simulink model "practica15sim"  (R2015a)
settings: Solver=ode45  StartTime=0.0  StopTime=30  RelTol=1e-3
settings Model: Creator=Sala8  LastModifiedBy=Sala7

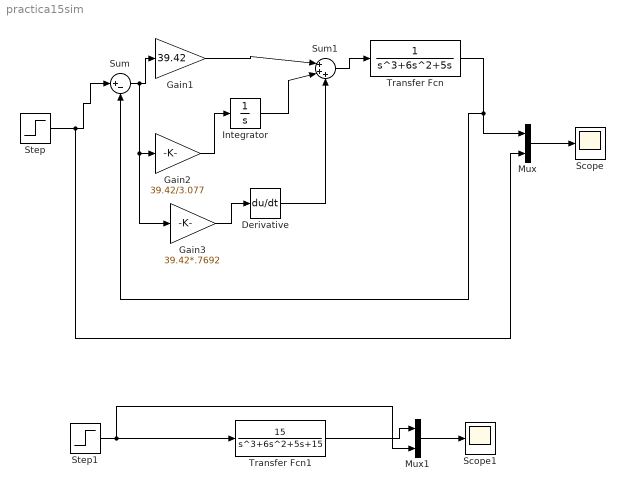
== system practica15sim ==
  Derivative : Derivative
  Gain1 : Gain  Gain=39.42
  Gain2 : Gain  Gain=39.42/3.077
  Gain3 : Gain  Gain=39.42*.7692
  Integrator : Integrator
  Mux : Mux  Inputs=2
  Mux1 : Mux  Inputs=2
  Scope : Scope
  Scope1 : Scope
  Step : Step  Time=0  SampleTime=0
  Step1 : Step  Time=0  SampleTime=0
  Sum : Sum  Inputs=|+-
  Sum1 : Sum  Inputs=|+++
  Transfer Fcn : TransferFcn  Denominator=[1 6 5 0]
  Transfer Fcn1 : TransferFcn  Numerator=[15]  Denominator=[1 6 5 15]
  wires:
  Step/1 -> Mux/2, Sum/1
  Mux/1 -> Scope/1
  Transfer Fcn/1 -> Sum/2, Mux/1
  Sum/1 -> Gain3/1, Gain2/1, Gain1/1
  Gain2/1 -> Integrator/1
  Gain1/1 -> Sum1/1
  Sum1/1 -> Transfer Fcn/1
  Step1/1 -> Transfer Fcn1/1, Mux1/2
  Mux1/1 -> Scope1/1
  Transfer Fcn1/1 -> Mux1/1
  Integrator/1 -> Sum1/2
  Gain3/1 -> Derivative/1
  Derivative/1 -> Sum1/3
